simulink model "real_control"  (R2023b)
settings: Solver=FixedStepDiscrete  StartTime=0.0  StopTime=inf  MaxStep=0.005  RelTol=1e-3  EnableMultiTasking=on
libraries: px4lib x2, px4uORBlib x1
settings Model: ExtModeTrigDuration=10  Creator=UAV2  LastModifiedBy=UAV2
settings SolverCC: PositivePriorityOrder=on
settings OptimizationCC: EnhancedBackFolding=on  PassReuseOutputArgsAs=Individual arguments  ZeroExternalMemoryAtStartup=off  ZeroInternalMemoryAtStartup=off  MaxStackSize=64  OptimizeBlockOrder=speed  DifferentSizesBufferReuse=on  OptimizationCustomize=off  EfficientTunableParamExpr=on
settings DebuggingCC: ParameterTunabilityLossMsg=error
settings HardwareCC: ProdBitPerPointer=32  ProdBitPerSizeT=32  ProdBitPerPtrDiffT=32  ProdLargestAtomicInteger=Long  ProdLargestAtomicFloat=Double  ProdWordSize=32  ProdLongLongMode=on  ProdHWDeviceType=ARM Compatible->ARM Cortex
settings SFSimCC: MATLABDynamicMemAlloc=off  SimTargetLang=C++
settings RTWCC: Description=Embedded Coder  SystemTargetFile=ert.tlc  HardwareBoard=PX4 Pixhawk 4  TLCOptions="-aInlineSetEventsForThisBaseRateFcn=TLC_FALSE -aSuppressMultiTaskScheduler=TLC_FALSE  -aRateBasedStepFcn=0"  TemplateMakefile=ert_default_tmf  Toolchain=GNU Tools for PX4 Autopilots  TargetLang=C++
settings CodeAppCC: ForceParamTrailComments=on  IgnoreCustomStorageClasses=off  OperatorAnnotations=on  SimulinkDataObjDesc=on  SFDataObjDesc=on  InsertBlockDesc=on
settings ERTTargetCC: ExtModeTransport=3  ExtModeStaticAlloc=on  ExtModeStaticAllocSize=1024  ExtModeMexFile=ext_xcp  ExtModeIntrfLevel=Level2 - Open

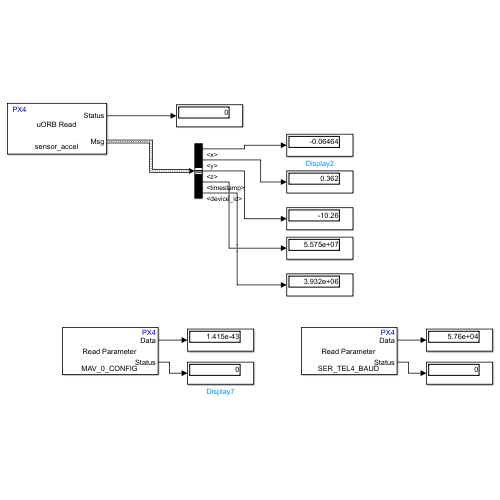
[thumbnail: Simulink's stored preview of the top-level diagram]
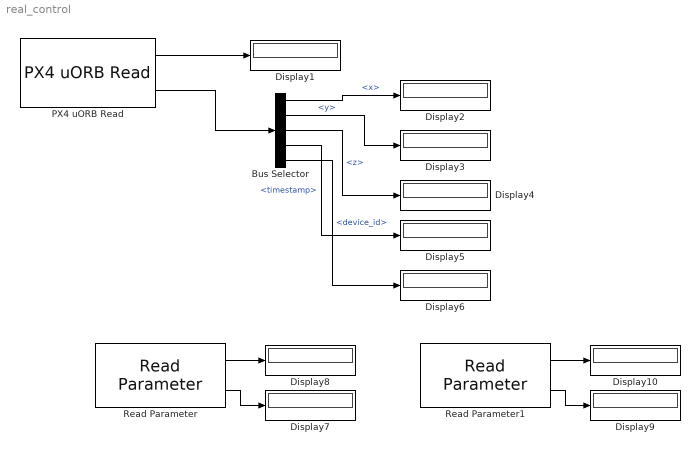
== system real_control ==
  Bus Selector : BusSelector  OutputSignals=x,y,z,timestamp,device_id
  Display{1..10} (10 alike) : Display
  PX4 uORB Read : px4uORBlib/PX4 uORB Read  uORBTopic=sensor_accel  selectInstance=sensor_accel  SampleTime=-1  BlockingMode=off  BlockTimeout=1e-3
  Read Parameter : px4lib/Read Parameter  ParameterName=MAV_0_CONFIG  DataType=FLOAT  SampleTime=0.5
  Read Parameter1 : px4lib/Read Parameter  ParameterName=SER_TEL4_BAUD  DataType=INT32  SampleTime=0.5
  wires:
  PX4 uORB Read/1 -> Display1/1
  PX4 uORB Read/2 -> Bus Selector/1
  Bus Selector/1 -> Display2/1  "<x>"
  Bus Selector/2 -> Display3/1  "<y>"
  Bus Selector/3 -> Display4/1  "<z>"
  Bus Selector/4 -> Display5/1  "<timestamp>"
  Bus Selector/5 -> Display6/1  "<device_id>"
  Read Parameter/2 -> Display7/1
  Read Parameter/1 -> Display8/1
  Read Parameter1/1 -> Display10/1
  Read Parameter1/2 -> Display9/1
